simulink model "Sim1"  (R2018a)
settings: Solver=ode4  StartTime=0.0  StopTime=10.0  FixedStep=1e-2  RelTol=1e-3
values from neighbouring files (symbols this model uses):
  K = 1/(R*C)    (= 1)    [s1.m]
  WPC = 4    [s1.m]    (also in s2.m = WPCa(:,:,2); s3.m = 1000)
settings Model: Creator=Igor  LastModifiedBy=Igor

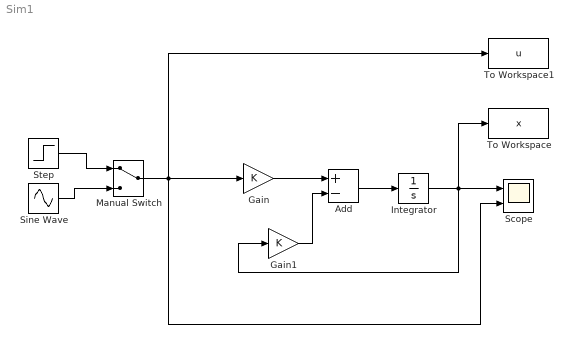
== system Sim1 ==
  Add : Sum  Inputs=+-
  Gain : Gain  Gain=K
  Gain1 : Gain  Gain=K
  Integrator : Integrator  InitialCondition=WPC
  Manual Switch : ManualSwitch
  Scope : Scope  NumInputPorts=2
  Sine Wave : Sin  SampleTime=0
  Step : Step  After=0  SampleTime=0
  To Workspace : ToWorkspace  VariableName=x  SampleTime=-1
  To Workspace1 : ToWorkspace  VariableName=u  SampleTime=-1
  wires:
  Step/1 -> Manual Switch/1
  Sine Wave/1 -> Manual Switch/2
  Manual Switch/1 -> To Workspace1/1, Scope/2, Gain/1
  Add/1 -> Integrator/1
  Integrator/1 -> Gain1/1, Scope/1, To Workspace/1
  Gain/1 -> Add/1
  Gain1/1 -> Add/2
